simulink model "simulink_sfbk"  (R2019b)
settings: Solver=ode4  StartTime=0.0  StopTime=4  FixedStep=0.01  RelTol=1e-3
values from neighbouring files (symbols this model uses):
  A = [0 1 0 0 ... (first row only)    [following.m]    (also in following2.m; observer.m; opt_servo.m; optimal_care.m = [0 1)
  B = [0 ... (first row only)    [following.m]    (also in following2.m; observer.m; opt_servo.m; optimal_care.m)
  K = -acker(A,B,p)    [following.m]    (also in following2.m = Ke(1:4); observer.m; opt_servo.m = -inv(Re)*B'*P11; optimal_care.m = -inv(R)*B'*P)
  x0 = zeros(4,1)    [following.m]    (also in following2.m; observer.m = [-0.5 0 0.5 0]'; opt_servo.m = [ 0 0 0.25 0 ]'; optimal_care.m = [1)
settings Model: Creator=shohei  LastModifiedBy=shohei

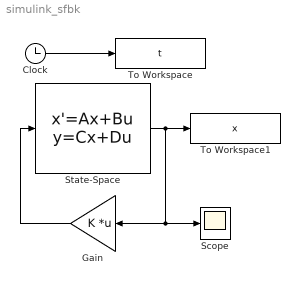
== system simulink_sfbk ==
  Clock : Clock
  Gain : Gain  Gain=K  Multiplication=Matrix(K*u)
  Scope : Scope
  State-Space : StateSpace  A=A  B=B  C=eye(2)  D=zeros(2,1)  InitialCondition=x0
  To Workspace : ToWorkspace  VariableName=t  SampleTime=-1
  To Workspace1 : ToWorkspace  VariableName=x  SampleTime=-1
  wires:
  Clock/1 -> To Workspace/1
  State-Space/1 -> Scope/1, Gain/1, To Workspace1/1
  Gain/1 -> State-Space/1
